simulink model "pointmass_param_mpc"  (Simulink 8.3)
settings: Solver=ode4  StartTime=0.0  StopTime=200  RelTol=1e-3
values from neighbouring files (symbols this model uses):
  A = [1 dt 0.5*dt*dt ... (first row only)    [mpc_parametric_setup.m]
  B = [0.5*dt*dt ... (first row only)    [mpc_parametric_setup.m]
  dt = 0.25    [mpc_parametric_setup.m]
  R = diag([5])    [mpc_parametric_setup.m]
libraries: softmpc x1, simulink x1
settings Model: Creator=aeagr  LastModifiedBy=aeagr
settings OptimizationCC: ExpressionDepthLimit=2147483647
settings DebuggingCC: FcnCallInpInsideContextMsg=EnableAllAsWarning

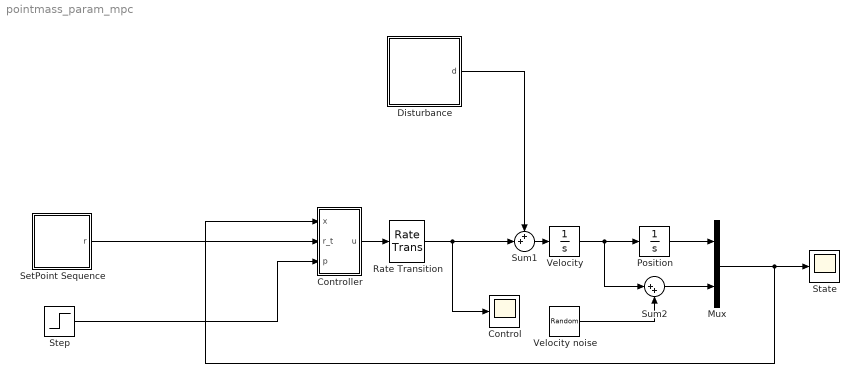
== system pointmass_param_mpc ==
  Control : Scope
      settings: TimeRange=240  YMin=-0.4  YMax=0.35
  Controller : Subsystem  TreatAsAtomicUnit=on  SystemSampleTime=dt
  Disturbance : Subsystem
  Mux : Mux  Inputs=2
  Position : Integrator
  Rate Transition : RateTransition
  SetPoint Sequence : Subsystem
  State : Scope
      settings: TimeRange=200  YMin=-1  YMax=14
  Step : Step  Time=100  Before=0.15  After=0  SampleTime=0
  Sum1 : Sum  Inputs=++|
  Sum2 : Sum  Inputs=|++
  Velocity : Integrator
  Velocity noise : RandomNumber  Variance=0.000000001  SampleTime=dt
  wires:
  Velocity/1 -> Position/1, Sum2/1
  Mux/1 -> Controller/1(x), State/1
  Position/1 -> Mux/1
  Sum1/1 -> Velocity/1
  Sum2/1 -> Mux/2
  Velocity noise/1 -> Sum2/2
  Disturbance/1(d) -> Sum1/1
  SetPoint Sequence/1(r) -> Controller/2(r_t)
  Step/1 -> Controller/3(p)
  Controller/1(u) -> Rate Transition/1
  Rate Transition/1 -> Control/1, Sum1/2

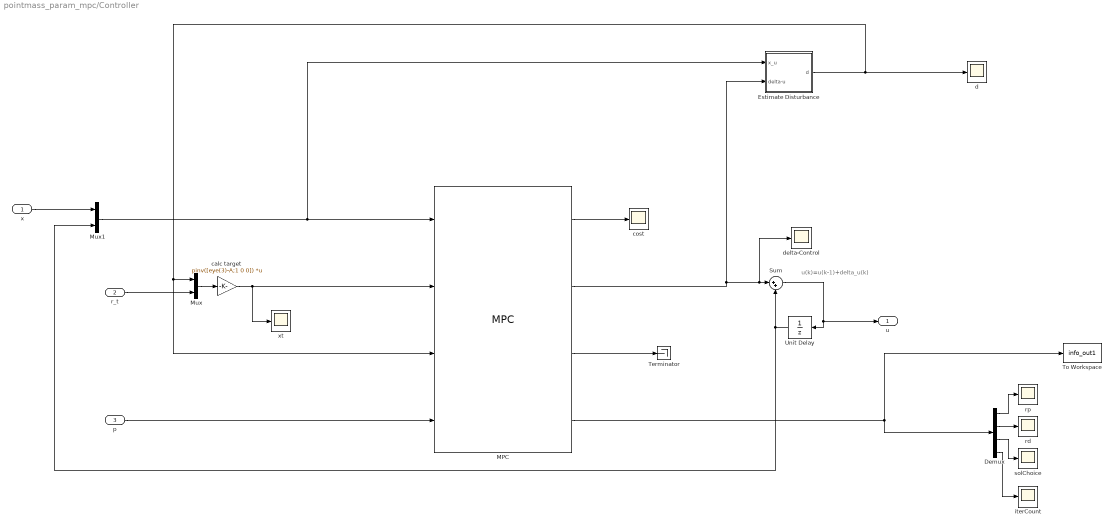
== system pointmass_param_mpc/Controller ==
  note: u(k)=u(k-1)+delta_u(k)
  x : Inport
  r_t : Inport  Port=2
  p : Inport  Port=3
  Demux : Demux
  Estimate Disturbance : Subsystem
  MPC : softmpc/MPC  A=A  B=B  T=6  dt=-1  Q=Q  R=R  Qf=Qf  qv=q  rv=r  qfv=qf  Fx=Fx  Fu=Fu  Fp=Fp  f=f  Fxs=Fxs  Fus=Fus  Fps=Fps  fs=fs  Fxf=Fxf  Fpf=Fpf  ff=ff  Ef=Ef  Ed=Ed  e=ef  consAllBox=on  numNewton=5  kappa=0.005
  Mux : Mux  Inputs=2
  Mux1 : Mux  Inputs=2
  Sum : Sum  Inputs=|++
  Terminator : Terminator
  To Workspace : ToWorkspace  VariableName=info_out1  SampleTime=-1
  Unit Delay : UnitDelay  SampleTime=-1
  calc target : Gain  Gain=pinv([eye(3)-A;1 0 0])  Multiplication=Matrix(K*u)
  cost : Scope
      settings: YMin=-0.25  YMax=2.5  SaveName=ScopeData10
  d : Scope
      settings: YMin=-0.00025  YMax=0.002  SaveName=ScopeData11
  delta-Control : Scope
      settings: TimeRange=240  YMin=-0.4  YMax=0.35  SaveName=ScopeData2
  iterCount : Scope
      settings: TimeRange=200  YMin=0  YMax=25  SaveName=ScopeData12
  rd : Scope
      settings: YMin=0  YMax=13  SaveName=ScopeData13
  rp : Scope
      settings: YMin=1.65436e-24  YMax=2.75e-08  SaveName=ScopeData14
  solChoice : Scope
      settings: YMin=0.95  YMax=1.05  SaveName=ScopeData15
  xt : Scope
      settings: YMin=-0.25  YMax=2.5  SaveName=ScopeData16
  u : Outport
  wires:
  Sum/1 -> u/1, Unit Delay/1
  MPC/2 -> Sum/1, delta-Control/1, Estimate Disturbance/2(delta-u)
  Unit Delay/1 -> Sum/2, Mux1/2
  Mux1/1 -> MPC/1, Estimate Disturbance/1(x_u)
  Demux/1 -> rp/1
  Demux/2 -> rd/1
  Demux/3 -> solChoice/1
  Estimate Disturbance/1(d) -> MPC/3, Mux/1, d/1
  Mux/1 -> calc target/1
  r_t/1 -> Mux/2
  calc target/1 -> MPC/2, xt/1
  Demux/4 -> iterCount/1
  p/1 -> MPC/4
  MPC/1 -> cost/1
  x/1 -> Mux1/1
  MPC/4 -> To Workspace/1, Demux/1
  MPC/3 -> Terminator/1

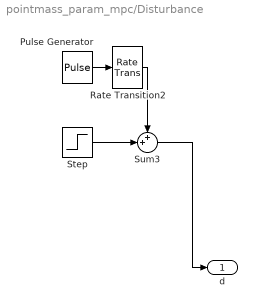
== system pointmass_param_mpc/Disturbance ==
  Pulse Generator : DiscretePulseGenerator  PulseType=Time based  Amplitude=0.1  Period=200  PhaseDelay=100
  Rate Transition2 : RateTransition
  Step : Step  Time=100  After=0.01  SampleTime=0
  Sum3 : Sum  Inputs=++|
  d : Outport
  wires:
  Step/1 -> Sum3/2
  Pulse Generator/1 -> Rate Transition2/1
  Sum3/1 -> d/1
  Rate Transition2/1 -> Sum3/1

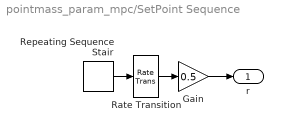
== system pointmass_param_mpc/SetPoint Sequence ==
  Gain : Gain  Gain=0.5
  Rate Transition : RateTransition
  Repeating Sequence Stair : simulink/Sources/Repeating Sequence Stair  OutValues=[1 0 2 0 3 0 4 0 5 0 6 0].'  tsamp=20  OutMin=[]  OutMax=[]  OutDataTypeStr=double  OutputDataTypeScalingMode=Specify via dialog  OutDataType=double  ConRadixGroup=Best Precision: Vector-wise  OutScaling=2^-12
  r : Outport
  wires:
  Repeating Sequence Stair/1 -> Rate Transition/1
  Rate Transition/1 -> Gain/1
  Gain/1 -> r/1

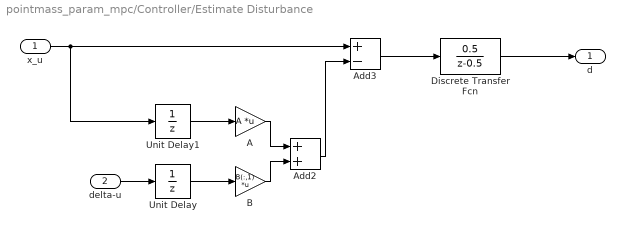
== system pointmass_param_mpc/Controller/Estimate Disturbance ==
  x_u : Inport
  delta-u : Inport  Port=2
  A : Gain  Gain=A  Multiplication=Matrix(K*u)
  Add2 : Sum
  Add3 : Sum  Inputs=+-
  B : Gain  Gain=B(:,1)  Multiplication=Matrix(K*u)
  Discrete Transfer Fcn : DiscreteTransferFcn  Numerator=[0.5]  Denominator=[1 -0.5]
  Unit Delay : UnitDelay  SampleTime=-1
  Unit Delay1 : UnitDelay  SampleTime=-1
  d : Outport
  wires:
  Unit Delay1/1 -> A/1
  Unit Delay/1 -> B/1
  A/1 -> Add2/1
  B/1 -> Add2/2
  Add2/1 -> Add3/2
  x_u/1 -> Unit Delay1/1, Add3/1
  delta-u/1 -> Unit Delay/1
  Add3/1 -> Discrete Transfer Fcn/1
  Discrete Transfer Fcn/1 -> d/1
